simulink model "Test_Pattern_Generator"  (R2013b)
settings: Solver=ode45  StartTime=0.0  StopTime=1500  RelTol=1e-3
InitFcn:
  | %% DSPBuilder Start
  | alt_dspbuilder_update_model(bdroot)
  | %% DSPBuilder End
libraries: allblocks_alteradspbuilder2 x106, simulink x4
(part 1 of 2)
settings Model: Creator=Given_Jiang  LastModifiedBy=Given_Jiang

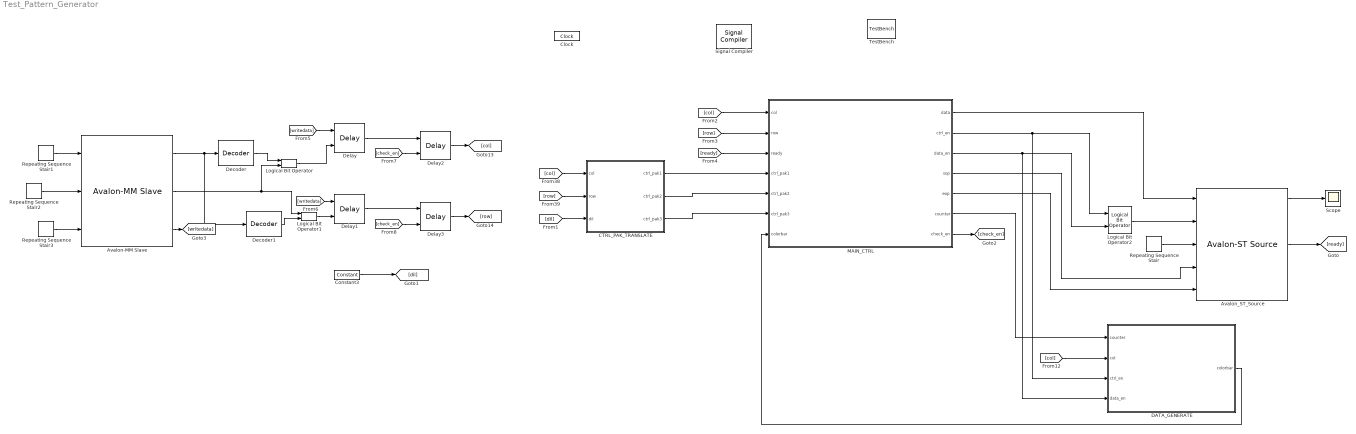
== system Test_Pattern_Generator ==
  Avalon-MM Slave : allblocks_alteradspbuilder2/Avalon-MM Slave  iofile=E:\FPGA\SOC\Quartus\quartus\dsp_builder\design\VIP_LIB\Test_Pattern_Generator\tb_Test_Pattern_Generator\Test%5FPattern%5FGenerator_Avalon-MM+Slave_address.salt,E:\FPGA\SOC\Quartus\quartus\dsp_builder\design\VIP_LIB\Test_Pattern_Generator\tb_Test_Pattern_Generator\Test%5FPattern%5FGenerator_Avalon-MM+Slave_write.salt,E:\FPGA\SOC\Quartus\quartus\dsp_builder\design\VIP_LIB\Test_Pattern_Generator\tb_Test_Pattern_Generator\Test%5FPattern%5FGenerator_Avalon-MM+Slave_writedata.salt,  SpecifyClock=off  addrWidth=2  addrAlignment=Dynamic  addrType=Write  BusType=Unsigned Integer  bwl=32  bwr=0  byteEnable=off  flowCtrl=off  pipeline=off  waitStateFormat=Fixed  readWaitStateCycles=0  writeWaitStateCycles=1  readLatencyFormat=Fixed  readLatencyCycles=0  burst=off  maxBurst=4  irq=off  receiveBeginTransfer=off  useChipSelect=off  externalType=Inferred  PORTTYPE=Output
  Avalon_ST_Source : allblocks_alteradspbuilder2/Avalon-ST Source  iofile=E:\FPGA\SOC\Quartus\quartus\dsp_builder\design\VIP_LIB\Test_Pattern_Generator\tb_Test_Pattern_Generator\Test%5FPattern%5FGenerator_Avalon%5FST%5FSource_data.capture,E:\FPGA\SOC\Quartus\quartus\dsp_builder\design\VIP_LIB\Test_Pattern_Generator\tb_Test_Pattern_Generator\Test%5FPattern%5FGenerator_Avalon%5FST%5FSource_valid.capture,E:\FPGA\SOC\Quartus\quartus\dsp_builder\design\VIP_LIB\Test_Pattern_Generator\tb_Test_Pattern_Generator\Test%5FPattern%5FGenerator_Avalon%5FST%5FSource_ready.salt,E:\FPGA\SOC\Quartus\quartus\dsp_builder\design\VIP_LIB\Test_Pattern_Generator\tb_Test_Pattern_Generator\Test%5FPattern%5FGenerator_Avalon%5FST%5FSource_startofpacket.capture,E:\FPGA\SOC\Quartus\quartus\dsp_builder\design\VIP_LIB\Test_Pattern_Generator\tb_Test_Pattern_Generator\Test%5FPattern%5FGenerator_Avalon%5FST%5FSource_endofpacket.capture,  SpecifyClock=off  BusType=Unsigned Integer  bwl=24  bwr=0  symbolWidth=8  symbolsPerBeat=3  numOfChannels=0  numOfErrorDescriptors=0  endOfPacket=on  startOfPacket=on  empty=off  readyLatency=1  externalType=Inferred  PORTTYPE=Input
  CTRL_PAK_TRANSLATE : Subsystem
  Clock : allblocks_alteradspbuilder2/Clock  ClockPeriod=7.5  ClockPeriodUnit=ns  SampleTime=1  ResetLatency=0  ResetRegisterCascadeDepth=0  SimulationStartCycle=5  PhaseOffset=0  Reset=aclr  ResetType=Active Low  Export=off
  Constant3 : allblocks_alteradspbuilder2/Constant  mask_cst=0  BusType=Signed Integer  bwl=4  bwr=0  roundMode=Truncate  satMode=Wrap  SpecifyClock=off  allowFloatingPointOverride=on  logOutputs=off  logFile=E:\FPGA\SOC\Quartus\quartus\dsp_builder\design\VIP_LIB\Test_Pattern_Generator\tb_Test_Pattern_Generator\Test%5FPattern%5FGenerator_Constant3.fixedpointlog
  DATA_GENERATE : Subsystem
  Decoder : allblocks_alteradspbuilder2/Decoder  BusType=Unsigned Integer  bwl=2  bwr=2  registered=on  pipeline_display=1  value=1
  Decoder1 : allblocks_alteradspbuilder2/Decoder  BusType=Unsigned Integer  bwl=2  bwr=2  registered=on  pipeline_display=1  value=2
  Delay : allblocks_alteradspbuilder2/Delay  pipeline=1  pipeline_display=1  ClockPhase=1  use_ena=on  use_sclr=off  allowFloatingPointOverride=on  logOutputs=off  logFile=E:\FPGA\SOC\Quartus\quartus\dsp_builder\design\VIP_LIB\Test_Pattern_Generator\tb_Test_Pattern_Generator\Test%5FPattern%5FGenerator_Delay.fixedpointlog  use_init=on  reset_value=32
  Delay1 : allblocks_alteradspbuilder2/Delay  pipeline=1  pipeline_display=1  ClockPhase=1  use_ena=on  use_sclr=off  allowFloatingPointOverride=on  logOutputs=off  logFile=E:\FPGA\SOC\Quartus\quartus\dsp_builder\design\VIP_LIB\Test_Pattern_Generator\tb_Test_Pattern_Generator\Test%5FPattern%5FGenerator_Delay1.fixedpointlog  use_init=on  reset_value=32
  Delay2 : allblocks_alteradspbuilder2/Delay  pipeline=1  pipeline_display=1  ClockPhase=1  use_ena=on  use_sclr=off  allowFloatingPointOverride=on  logOutputs=off  logFile=E:\FPGA\SOC\Quartus\quartus\dsp_builder\design\VIP_LIB\Test_Pattern_Generator\tb_Test_Pattern_Generator\Test%5FPattern%5FGenerator_Delay2.fixedpointlog  use_init=on  reset_value=32
  Delay3 : allblocks_alteradspbuilder2/Delay  pipeline=1  pipeline_display=1  ClockPhase=1  use_ena=on  use_sclr=off  allowFloatingPointOverride=on  logOutputs=off  logFile=E:\FPGA\SOC\Quartus\quartus\dsp_builder\design\VIP_LIB\Test_Pattern_Generator\tb_Test_Pattern_Generator\Test%5FPattern%5FGenerator_Delay3.fixedpointlog  use_init=on  reset_value=32
  Logical Bit Operator : allblocks_alteradspbuilder2/Logical Bit Operator  LogicalOperator=AND  user_inputs=2  pipeline_display=0
  Logical Bit Operator1 : allblocks_alteradspbuilder2/Logical Bit Operator  LogicalOperator=AND  user_inputs=2  pipeline_display=0
  Logical Bit Operator2 : allblocks_alteradspbuilder2/Logical Bit Operator  LogicalOperator=OR  user_inputs=2  pipeline_display=0
  MAIN_CTRL : Subsystem
  Repeating Sequence Stair : simulink/Sources/Repeating Sequence Stair  OutValues=[0 1 1 1 1 1 1].'  tsamp=-1  OutMin=[]  OutMax=[]  OutDataTypeStr=double  OutputDataTypeScalingMode=double  OutDataType=fixdt(0,8)  ConRadixGroup=Best Precision: Vector-wise  OutScaling=2^-12
  Repeating Sequence Stair1 : simulink/Sources/Repeating Sequence Stair  OutValues=[1].'  tsamp=-1  OutMin=[]  OutMax=[]  OutDataTypeStr=double  OutputDataTypeScalingMode=double  OutDataType=fixdt(0,8)  ConRadixGroup=Best Precision: Vector-wise  OutScaling=2^-12
  Repeating Sequence Stair2 : simulink/Sources/Repeating Sequence Stair  OutValues=[1].'  tsamp=-1  OutMin=[]  OutMax=[]  OutDataTypeStr=double  OutputDataTypeScalingMode=double  OutDataType=fixdt(0,8)  ConRadixGroup=Best Precision: Vector-wise  OutScaling=2^-12
  Repeating Sequence Stair3 : simulink/Sources/Repeating Sequence Stair  OutValues=[255].'  tsamp=-1  OutMin=[]  OutMax=[]  OutDataTypeStr=double  OutputDataTypeScalingMode=double  OutDataType=fixdt(0,8)  ConRadixGroup=Best Precision: Vector-wise  OutScaling=2^-12
  Scope : Scope
  Signal Compiler : allblocks_alteradspbuilder2/Signal Compiler  DeviceFamily=Cyclone V  DeviceName=AUTO  DisableEarlyHDLGeneration=off  EnableSignalTap=off  SignalTapDepth=128  UseBoardBlock=off  StpUseDefaultClock=on  StpClock=Clock  ExportDir=E:\FPGA\SOC\Quartus\quartus\dsp_builder
  TestBench : allblocks_alteradspbuilder2/TestBench  enable=on  advancedMode=on  modelSimGui=off  maxDisplayErrors=10  mismatchErrorLevel=Error  simdatafile=E:\FPGA\SOC\Quartus\quartus\dsp_builder\design\VIP_LIB\Test_Pattern_Generator\tb_Test_Pattern_Generator\Test_Pattern_Generator.simdata.tcl
  wires:
  Avalon_ST_Source/3 -> [ready]
  Logical Bit Operator2/1 -> Avalon_ST_Source/2
  MAIN_CTRL/4(sop) -> Avalon_ST_Source/4
  MAIN_CTRL/5(eop) -> Avalon_ST_Source/5
  [row] -> CTRL_PAK_TRANSLATE/2(row)
  [col] -> CTRL_PAK_TRANSLATE/1(col)
  [dil] -> CTRL_PAK_TRANSLATE/3(dil)
  Constant3/1 -> [dil]
  [col] -> MAIN_CTRL/1(col)
  [row] -> MAIN_CTRL/2(row)
  [ready] -> MAIN_CTRL/3(ready)
  CTRL_PAK_TRANSLATE/1(ctrl_pak1) -> MAIN_CTRL/4(ctrl_pak1)
  CTRL_PAK_TRANSLATE/2(ctrl_pak2) -> MAIN_CTRL/5(ctrl_pak2)
  CTRL_PAK_TRANSLATE/3(ctrl_pak3) -> MAIN_CTRL/6(ctrl_pak3)
  [col] -> DATA_GENERATE/2(col)
  DATA_GENERATE/1(colorbar) -> MAIN_CTRL/7(colorbar)
  MAIN_CTRL/6(counter) -> DATA_GENERATE/1(counter)
  MAIN_CTRL/3(data_en) -> DATA_GENERATE/4(data_en), Logical Bit Operator2/2
  MAIN_CTRL/2(ctrl_en) -> DATA_GENERATE/3(ctrl_en), Logical Bit Operator2/1
  MAIN_CTRL/1(data) -> Avalon_ST_Source/1
  Repeating Sequence Stair/1 -> Avalon_ST_Source/3
  MAIN_CTRL/7(check_en) -> [check_en]
  Logical Bit Operator/1 -> Delay/2
  Delay/1 -> Delay2/1
  [check_en] -> Delay2/2
  [check_en] -> Delay3/2
  Delay1/1 -> Delay3/1
  Delay2/1 -> [col]
  Delay3/1 -> [row]
  Avalon_ST_Source/1 -> Scope/1
  Repeating Sequence Stair1/1 -> Avalon-MM Slave/1
  Repeating Sequence Stair3/1 -> Avalon-MM Slave/3
  Avalon-MM Slave/1 -> Decoder1/1, Decoder/1
  Decoder/1 -> Logical Bit Operator/1
  Avalon-MM Slave/2 -> Logical Bit Operator1/1, Logical Bit Operator/2
  Decoder1/1 -> Logical Bit Operator1/2
  Logical Bit Operator1/1 -> Delay1/2
  Avalon-MM Slave/3 -> [writedata]
  [writedata] -> Delay/1
  [writedata] -> Delay1/1
  Repeating Sequence Stair2/1 -> Avalon-MM Slave/2

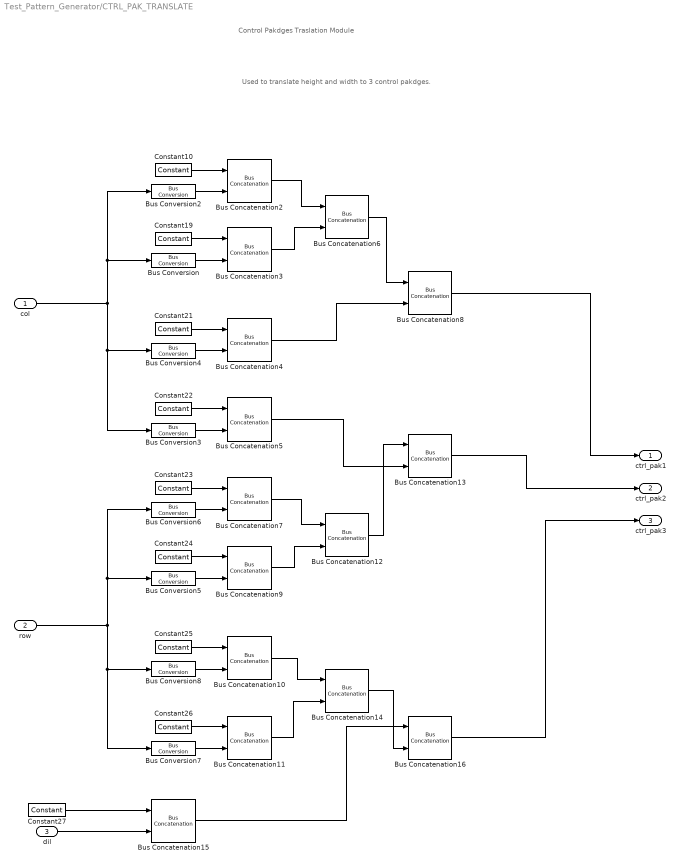
== system Test_Pattern_Generator/CTRL_PAK_TRANSLATE ==
  note: Used to translate height and width to 3 control pakdges.
  note: Control Pakdges Traslation Module
  col : Inport
  row : Inport  Port=2
  dil : Inport  Port=3
  Bus Concatenation{2..5,7,9..11,15} (9 alike) : allblocks_alteradspbuilder2/Bus Concatenation  isSigned=off  awidth=4  bwidth=4  pipeline_display=0
  Bus Concatenation12 : allblocks_alteradspbuilder2/Bus Concatenation  isSigned=off  awidth=8  bwidth=8  pipeline_display=0
  Bus Concatenation13 : allblocks_alteradspbuilder2/Bus Concatenation  isSigned=off  awidth=16  bwidth=8  pipeline_display=0
  Bus Concatenation14 : allblocks_alteradspbuilder2/Bus Concatenation  isSigned=off  awidth=8  bwidth=8  pipeline_display=0
  Bus Concatenation16 : allblocks_alteradspbuilder2/Bus Concatenation  isSigned=off  awidth=8  bwidth=16  pipeline_display=0
  Bus Concatenation6 : allblocks_alteradspbuilder2/Bus Concatenation  isSigned=off  awidth=8  bwidth=8  pipeline_display=0
  Bus Concatenation8 : allblocks_alteradspbuilder2/Bus Concatenation  isSigned=off  awidth=16  bwidth=8  pipeline_display=0
  Bus Conversion : allblocks_alteradspbuilder2/Bus Conversion  BusType=Unsigned Integer  ibwl=16  ibwr=1  bwl=4  bwr=1  bitToConnectToOutputLSB=8  round=off  saturate=off  pipeline_display=0
  Bus Conversion2 : allblocks_alteradspbuilder2/Bus Conversion  BusType=Unsigned Integer  ibwl=16  ibwr=1  bwl=4  bwr=1  bitToConnectToOutputLSB=4  round=off  saturate=off  pipeline_display=0
  Bus Conversion3 : allblocks_alteradspbuilder2/Bus Conversion  BusType=Unsigned Integer  ibwl=16  ibwr=1  bwl=4  bwr=1  bitToConnectToOutputLSB=0  round=off  saturate=off  pipeline_display=0
  Bus Conversion4 : allblocks_alteradspbuilder2/Bus Conversion  BusType=Unsigned Integer  ibwl=16  ibwr=1  bwl=4  bwr=1  bitToConnectToOutputLSB=12  round=off  saturate=off  pipeline_display=0
  Bus Conversion5 : allblocks_alteradspbuilder2/Bus Conversion  BusType=Unsigned Integer  ibwl=16  ibwr=1  bwl=4  bwr=1  bitToConnectToOutputLSB=12  round=off  saturate=off  pipeline_display=0
  Bus Conversion6 : allblocks_alteradspbuilder2/Bus Conversion  BusType=Unsigned Integer  ibwl=16  ibwr=1  bwl=4  bwr=1  bitToConnectToOutputLSB=8  round=off  saturate=off  pipeline_display=0
  Bus Conversion7 : allblocks_alteradspbuilder2/Bus Conversion  BusType=Unsigned Integer  ibwl=16  ibwr=1  bwl=4  bwr=1  bitToConnectToOutputLSB=4  round=off  saturate=off  pipeline_display=0
  Bus Conversion8 : allblocks_alteradspbuilder2/Bus Conversion  BusType=Unsigned Integer  ibwl=16  ibwr=1  bwl=4  bwr=1  bitToConnectToOutputLSB=0  round=off  saturate=off  pipeline_display=0
  Constant10 : allblocks_alteradspbuilder2/Constant  mask_cst=0  BusType=Signed Integer  bwl=4  bwr=0  roundMode=Truncate  satMode=Wrap  SpecifyClock=off  allowFloatingPointOverride=on  logOutputs=off  logFile=E:\FPGA\SOC\Quartus\quartus\dsp_builder\design\VIP_LIB\Test_Pattern_Generator\tb_Test_Pattern_Generator\Test%5FPattern%5FGenerator_CTRL%5FPAK%5FTRANSLATE_Constant10.fixedpointlog
  Constant19 : allblocks_alteradspbuilder2/Constant  mask_cst=0  BusType=Signed Integer  bwl=4  bwr=0  roundMode=Truncate  satMode=Wrap  SpecifyClock=off  allowFloatingPointOverride=on  logOutputs=off  logFile=E:\FPGA\SOC\Quartus\quartus\dsp_builder\design\VIP_LIB\Test_Pattern_Generator\tb_Test_Pattern_Generator\Test%5FPattern%5FGenerator_CTRL%5FPAK%5FTRANSLATE_Constant19.fixedpointlog
  Constant21 : allblocks_alteradspbuilder2/Constant  mask_cst=0  BusType=Signed Integer  bwl=4  bwr=0  roundMode=Truncate  satMode=Wrap  SpecifyClock=off  allowFloatingPointOverride=on  logOutputs=off  logFile=E:\FPGA\SOC\Quartus\quartus\dsp_builder\design\VIP_LIB\Test_Pattern_Generator\tb_Test_Pattern_Generator\Test%5FPattern%5FGenerator_CTRL%5FPAK%5FTRANSLATE_Constant21.fixedpointlog
  Constant22 : allblocks_alteradspbuilder2/Constant  mask_cst=0  BusType=Signed Integer  bwl=4  bwr=0  roundMode=Truncate  satMode=Wrap  SpecifyClock=off  allowFloatingPointOverride=on  logOutputs=off  logFile=E:\FPGA\SOC\Quartus\quartus\dsp_builder\design\VIP_LIB\Test_Pattern_Generator\tb_Test_Pattern_Generator\Test%5FPattern%5FGenerator_CTRL%5FPAK%5FTRANSLATE_Constant22.fixedpointlog
  Constant23 : allblocks_alteradspbuilder2/Constant  mask_cst=0  BusType=Signed Integer  bwl=4  bwr=0  roundMode=Truncate  satMode=Wrap  SpecifyClock=off  allowFloatingPointOverride=on  logOutputs=off  logFile=E:\FPGA\SOC\Quartus\quartus\dsp_builder\design\VIP_LIB\Test_Pattern_Generator\tb_Test_Pattern_Generator\Test%5FPattern%5FGenerator_CTRL%5FPAK%5FTRANSLATE_Constant23.fixedpointlog
  Constant24 : allblocks_alteradspbuilder2/Constant  mask_cst=0  BusType=Signed Integer  bwl=4  bwr=0  roundMode=Truncate  satMode=Wrap  SpecifyClock=off  allowFloatingPointOverride=on  logOutputs=off  logFile=E:\FPGA\SOC\Quartus\quartus\dsp_builder\design\VIP_LIB\Test_Pattern_Generator\tb_Test_Pattern_Generator\Test%5FPattern%5FGenerator_CTRL%5FPAK%5FTRANSLATE_Constant24.fixedpointlog
  Constant25 : allblocks_alteradspbuilder2/Constant  mask_cst=0  BusType=Signed Integer  bwl=4  bwr=0  roundMode=Truncate  satMode=Wrap  SpecifyClock=off  allowFloatingPointOverride=on  logOutputs=off  logFile=E:\FPGA\SOC\Quartus\quartus\dsp_builder\design\VIP_LIB\Test_Pattern_Generator\tb_Test_Pattern_Generator\Test%5FPattern%5FGenerator_CTRL%5FPAK%5FTRANSLATE_Constant25.fixedpointlog
  Constant26 : allblocks_alteradspbuilder2/Constant  mask_cst=0  BusType=Signed Integer  bwl=4  bwr=0  roundMode=Truncate  satMode=Wrap  SpecifyClock=off  allowFloatingPointOverride=on  logOutputs=off  logFile=E:\FPGA\SOC\Quartus\quartus\dsp_builder\design\VIP_LIB\Test_Pattern_Generator\tb_Test_Pattern_Generator\Test%5FPattern%5FGenerator_CTRL%5FPAK%5FTRANSLATE_Constant26.fixedpointlog
  Constant27 : allblocks_alteradspbuilder2/Constant  mask_cst=0  BusType=Signed Integer  bwl=4  bwr=0  roundMode=Truncate  satMode=Wrap  SpecifyClock=off  allowFloatingPointOverride=on  logOutputs=off  logFile=E:\FPGA\SOC\Quartus\quartus\dsp_builder\design\VIP_LIB\Test_Pattern_Generator\tb_Test_Pattern_Generator\Test%5FPattern%5FGenerator_CTRL%5FPAK%5FTRANSLATE_Constant27.fixedpointlog
  ctrl_pak1 : Outport
  ctrl_pak2 : Outport  Port=2
  ctrl_pak3 : Outport  Port=3
  wires:
  col/1 -> Bus Conversion3/1, Bus Conversion4/1, Bus Conversion2/1, Bus Conversion/1
  Bus Conversion2/1 -> Bus Concatenation2/2
  Constant10/1 -> Bus Concatenation2/1
  Constant19/1 -> Bus Concatenation3/1
  Bus Conversion/1 -> Bus Concatenation3/2
  Constant21/1 -> Bus Concatenation4/1
  Bus Conversion4/1 -> Bus Concatenation4/2
  Constant22/1 -> Bus Concatenation5/1
  Bus Conversion3/1 -> Bus Concatenation5/2
  Bus Concatenation3/1 -> Bus Concatenation6/2
  Bus Concatenation4/1 -> Bus Concatenation8/2
  Bus Concatenation6/1 -> Bus Concatenation8/1
  row/1 -> Bus Conversion7/1, Bus Conversion8/1, Bus Conversion6/1, Bus Conversion5/1
  Bus Conversion6/1 -> Bus Concatenation7/2
  Constant23/1 -> Bus Concatenation7/1
  Constant24/1 -> Bus Concatenation9/1
  Bus Conversion5/1 -> Bus Concatenation9/2
  Constant25/1 -> Bus Concatenation10/1
  Bus Conversion8/1 -> Bus Concatenation10/2
  Constant26/1 -> Bus Concatenation11/1
  Bus Conversion7/1 -> Bus Concatenation11/2
  Bus Concatenation7/1 -> Bus Concatenation12/1
  Bus Concatenation9/1 -> Bus Concatenation12/2
  Bus Concatenation10/1 -> Bus Concatenation14/1
  Bus Concatenation11/1 -> Bus Concatenation14/2
  dil/1 -> Bus Concatenation15/2
  Constant27/1 -> Bus Concatenation15/1
  Bus Concatenation8/1 -> ctrl_pak1/1
  Bus Concatenation13/1 -> ctrl_pak2/1
  Bus Concatenation16/1 -> ctrl_pak3/1
  Bus Concatenation2/1 -> Bus Concatenation6/1
  Bus Concatenation5/1 -> Bus Concatenation13/2
  Bus Concatenation12/1 -> Bus Concatenation13/1
  Bus Concatenation15/1 -> Bus Concatenation16/1
  Bus Concatenation14/1 -> Bus Concatenation16/2

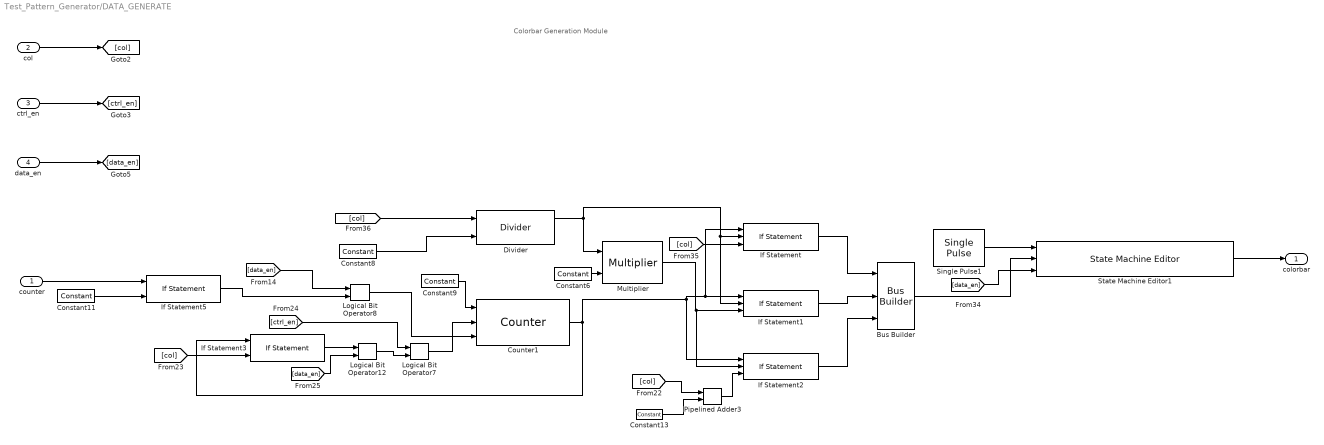
== system Test_Pattern_Generator/DATA_GENERATE ==
  note: Colorbar Generation Module
  counter : Inport
  col : Inport  Port=2
  ctrl_en : Inport  Port=3
  data_en : Inport  Port=4
  Bus Builder : allblocks_alteradspbuilder2/Bus Builder  BusType=Unsigned Integer  bwl=3  bwr=1  pipeline_display=0
  Constant11 : allblocks_alteradspbuilder2/Constant  mask_cst=4  BusType=Unsigned Integer  bwl=16  bwr=0  roundMode=Truncate  satMode=Wrap  SpecifyClock=off  allowFloatingPointOverride=on  logOutputs=off  logFile=E:\FPGA\SOC\Quartus\quartus\dsp_builder\design\VIP_LIB\Test_Pattern_Generator\tb_Test_Pattern_Generator\Test%5FPattern%5FGenerator_DATA%5FGENERATE_Constant11.fixedpointlog
  Constant13 : allblocks_alteradspbuilder2/Constant  mask_cst=1  BusType=Unsigned Integer  bwl=24  bwr=0  roundMode=Truncate  satMode=Wrap  SpecifyClock=off  allowFloatingPointOverride=on  logOutputs=off  logFile=E:\FPGA\SOC\Quartus\quartus\dsp_builder\design\VIP_LIB\Test_Pattern_Generator\tb_Test_Pattern_Generator\Test%5FPattern%5FGenerator_DATA%5FGENERATE_Constant13.fixedpointlog
  Constant6 : allblocks_alteradspbuilder2/Constant  mask_cst=2  BusType=Unsigned Integer  bwl=24  bwr=0  roundMode=Truncate  satMode=Wrap  SpecifyClock=off  allowFloatingPointOverride=on  logOutputs=off  logFile=E:\FPGA\SOC\Quartus\quartus\dsp_builder\design\VIP_LIB\Test_Pattern_Generator\tb_Test_Pattern_Generator\Test%5FPattern%5FGenerator_DATA%5FGENERATE_Constant6.fixedpointlog
  Constant8 : allblocks_alteradspbuilder2/Constant  mask_cst=3  BusType=Unsigned Integer  bwl=24  bwr=0  roundMode=Truncate  satMode=Wrap  SpecifyClock=off  allowFloatingPointOverride=on  logOutputs=off  logFile=E:\FPGA\SOC\Quartus\quartus\dsp_builder\design\VIP_LIB\Test_Pattern_Generator\tb_Test_Pattern_Generator\Test%5FPattern%5FGenerator_DATA%5FGENERATE_Constant8.fixedpointlog
  Constant9 : allblocks_alteradspbuilder2/Constant  mask_cst=1  BusType=Unsigned Integer  bwl=24  bwr=0  roundMode=Truncate  satMode=Wrap  SpecifyClock=off  allowFloatingPointOverride=on  logOutputs=off  logFile=E:\FPGA\SOC\Quartus\quartus\dsp_builder\design\VIP_LIB\Test_Pattern_Generator\tb_Test_Pattern_Generator\Test%5FPattern%5FGenerator_DATA%5FGENERATE_Constant9.fixedpointlog
  Counter1 : allblocks_alteradspbuilder2/Counter  BusType=Unsigned Integer  bwl=24  bwr=0  use_modulo=on  modulo=2^16  SpecifyClock=off  direction=Increment  use_sload=on  use_sset=off  svalue=1  use_clk_ena=off  use_ena=on  use_sclr=off  pipeline_display=1
  Divider : allblocks_alteradspbuilder2/Divider  BusType=Unsigned Integer  bwl=24  bwr=0  pipeline=0  pipeline_display=0  use_ena=off  use_aclr=off
  If Statement : allblocks_alteradspbuilder2/If Statement  user_inputs=3  if_expression=((a>0)&(a<b))|(a=c)  BusType=Unsigned Integer  bwl=24  bwr=0  pipeline_display=1  use_else_output=off  use_elseif_input=off
  If Statement1 : allblocks_alteradspbuilder2/If Statement  user_inputs=3  if_expression=((a>b)|(a=b))&(a<c)  BusType=Unsigned Integer  bwl=24  bwr=0  pipeline_display=1  use_else_output=off  use_elseif_input=off
  If Statement2 : allblocks_alteradspbuilder2/If Statement  user_inputs=3  if_expression=((a>b)|(a=b))&((a<c)|(a=c))  BusType=Unsigned Integer  bwl=24  bwr=0  pipeline_display=1  use_else_output=off  use_elseif_input=off
  If Statement3 : allblocks_alteradspbuilder2/If Statement  user_inputs=2  if_expression=a=b  BusType=Unsigned Integer  bwl=24  bwr=0  pipeline_display=1  use_else_output=off  use_elseif_input=off
  If Statement5 : allblocks_alteradspbuilder2/If Statement  user_inputs=2  if_expression=a>b  BusType=Unsigned Integer  bwl=24  bwr=0  pipeline_display=1  use_else_output=off  use_elseif_input=off
  Logical Bit Operator12 : allblocks_alteradspbuilder2/Logical Bit Operator  LogicalOperator=AND  user_inputs=2  pipeline_display=0
  Logical Bit Operator7 : allblocks_alteradspbuilder2/Logical Bit Operator  LogicalOperator=OR  user_inputs=2  pipeline_display=0
  Logical Bit Operator8 : allblocks_alteradspbuilder2/Logical Bit Operator  LogicalOperator=AND  user_inputs=2  pipeline_display=0
  Multiplier : allblocks_alteradspbuilder2/Multiplier  BusType=Unsigned Integer  bwl=24  bwr=0  pipeline=0  pipeline_display=0  allowFloatingPointOverride=on  logOutputs=off  logFile=E:\FPGA\SOC\Quartus\quartus\dsp_builder\design\VIP_LIB\Test_Pattern_Generator\tb_Test_Pattern_Generator\Test%5FPattern%5FGenerator_DATA%5FGENERATE_Multiplier.fixedpointlog  UseEqualInputWidth=on  bbwl=8  bbwr=0  FullResolution=on  OutputMsb=8  OutputLsb=0  OutputBwl=16  OutputBwr=16  UseDedicatedCircuitry=YES  use_ena=off  use_aclr=off
  Pipelined Adder3 : allblocks_alteradspbuilder2/Pipelined Adder  BusType=Unsigned Integer  bwl=24  bwr=0  pipeline=2  pipeline_display=2  AddSubDirection=SUB  use_cin=off  use_ovl=off  use_addsub=off  use_ena=off  use_aclr=off  or_aclr_inputs=on
  Single Pulse1 : allblocks_alteradspbuilder2/Single Pulse  signal_type=Step Down  impulse_width=1  delay=1  SpecifyClock=off  use_ena=off  use_sclr=off
  State Machine Editor1 : allblocks_alteradspbuilder2/State Machine Editor  entityName=StateMachineEditor1_import  use_dynamic_feedthrough_data=on  inNames=reset col_select data_en  inBwls=1 3 1  inBwrs="0  0  0"  inTypes=b s b  inDelayed="0  1  1"  outNames=data  outBwls=24  outBwrs=0  outTypes=s  n_input_port=3  n_output_port=1  array_clocks=clock  xmlmapfile=E:\FPGA\SOC\Quartus\quartus\dsp_builder\lib\SimgenCMap.xml  vofile=DSPBuilder_Test_Pattern_Generator_import\StateMachineEditor1.vo  use_systemC_model=off  is_megacore=off  smf_variation=|
      | /*                                                                         
      | WARNING: Do NOT edit the input and output ports in this file in a text     
      | editor if you plan to continue editing the block that represents it in     
      | the Block Editor! File corruption is VERY likely to occur.                 
      | Copyright (C) 1991-2013 Altera Corporation                                 
      | Your use of Altera Corporation's design tools, logic functions             
      | and other software and tools, and its AMPP partner logic                   
      | functions, and any output files from any of the foregoing                  
      | (including device programming or simulation files), and any                
      | associated documentation or information are expressly subject              
      | to the terms and conditions of the Altera Program License                  
      | Subscription Agreement, Altera MegaCore Function License                   
      | Agreement, or other applicable license agreement, including,               
      | without limitation, that your use is for the sole purpose of               
      | programming logic devices manufactured by Altera and sold by               
      | Altera or its authorized distributors.  Please refer to the                
      | applicable agreement for further details.                                  
      | Generated by Quartus II Version 13.1.0 Build 162 10/23/2013 SJ Full Version
      | Created on Sat Feb 07 15:51:54 2015                                        
      | */                                                                         
      | VERSION = "3.0";                                                           
      | HEADER                                                                     
      | (                                                                          
      | 	GENERAL{                                                                  
      | 		RMODE = "S";                                                             
      | 		RA_LEVEL = "H";                                                          
      | 		HOPT = "VHDL";                                                           
      | 	}                                                                         
      | 	SPORT{                                                                    
      | 		NAME = "clock";                                                          
      | 		PTYPE = "CI";                                                            
      | 		REG = "N";                                                               
      | 		OUTS = "N";                                                              
      | 	}                                                                         
      | 	SPORT{                                                                    
      | 		NAME = "reset";                                                          
      | 		PTYPE = "RI";                                                            
      | 		REG = "N";                                                               
      | 		OUTS = "N";                                                              
      | 	}                                                                         
      | 	SPORT{                                                                    
      | 		NAME = "col_select[2:0]";                                                
      | 		PTYPE = "OI";                                                            
      | 		REG = "N";                                                               
      | 		OUTS = "N";                                                              
      | 	}                                                                         
      | 	SPORT{                                                                    
      | 		NAME = "data_en";                                                        
      | 		PTYPE = "OI";                                                            
      | 		REG = "N";                                                               
      | 		OUTS = "N";                                                              
      | 	}                                                                         
      | 	SPORT{                                                                    
      | 		NAME = "data[23:0]";                                                     
      | 		PTYPE = "OU";                                                            
      | 		REG = "N";                                                               
      | 		OUTS = "C";                                                              
      | 	}                                                                         
      | 	STATE{                                                                    
      | 		NAME = "IDLE";                                                           
      | 		STYPE = "RE";                                                            
      | 		PT = (192,224);                                                          
      | 		OUTP = "data[23:0]";                                                     
      | 		OUT_VALUE = "0";                                                         
      | 		COND = "";                                                               
      | 	}                                                                         
      | 	STATE{                                                                    
      | 		NAME = "BLOCKA";                                                         
      | 		STYPE = "NR";                                                            
      | 		PT = (368,224);                                                          
      | 		OUTP = "data[23:0]";                                                     
      | 		OUT_VALUE = "255";                                                       
      | 		COND = "";                                                               
      | 	}                                                                         
      | 	STATE{                                                                    
      | 		NAME = "BLOCKB";                                                         
      | 		STYPE = "NR";                                                            
      | 		PT = (520,224);                                                          
      | 		OUTP = "data[23:0]";                                                     
      | 		OUT_VALUE = "65280";                                                     
      | 		COND = "";                                                               
      | 	}                                                                         
      | 	STATE{                                                                    
      | 		NAME = "BLOCKC";                                                         
      | 		STYPE = "NR";                                                            
      | 		PT = (680,224);                                                          
      | 		OUTP = "data[23:0]";                                                     
      | 		OUT_VALUE = "16711680";                                                  
      | 		COND = "";                                                               
      | 	}                                                                         
      | 	TRANS{                                                                    
      | 		SSTATE = "BLOCKC";                                                       
      | 		DSTATE = "IDLE";                                                         
      | 		EQ = "col_select==0";                                                    
      | 		PT = (689,268);                                                          
      | 		PT = (573,317);                                                          
      | 		PT = (364,317);                                                          
      | 		PT = (231,268);                                                          
      | 		PT = (468,327);                                                          
      | 	}                                                                         
      | 	TRANS{                                                                    
      | 		SSTATE = "IDLE";                                                         
      | 		DSTATE = "BLOCKA";                                                       
      | 		EQ = "(col_select==1)&(data_en==1)";                                     
      | 		PT = (241,248);                                                          
      | 		PT = (283,248);                                                          
      | 		PT = (325,248);                                                          
      | 		PT = (367,248);                                                          
      | 		PT = (304,258);                                                          
      | 	}                                                                         
      | 	TRANS{                                                                    
      | 		SSTATE = "BLOCKA";                                                       
      | 		DSTATE = "BLOCKB";                                                       
      | 		EQ = "(col_select==2)&(data_en==1)";                                     
      | 		PT = (417,248);                                                          
      | 		PT = (451,248);                                                          
      | 		PT = (485,248);                                                          
      | 		PT = (519,248);                                                          
      | 		PT = (468,258);                                                          
      | 	}                                                                         
      | 	TRANS{                                                                    
      | 		SSTATE = "BLOCKB";                                                       
      | 		DSTATE = "BLOCKC";                                                       
      | 		EQ = "(col_select==4)&(data_en==1)";                                     
      | 		PT = (569,248);                                                          
      | 		PT = (605,248);                                                          
      | 		PT = (642,248);                                                          
      | 		PT = (679,248);                                                          
      | 		PT = (601,249);                                                          
      | 	}                                                                         
      | 	TRANS{                                                                    
      | 		SSTATE = "IDLE";                                                         
      | 		DSTATE = "IDLE";                                                         
      | 		EQ = "col_select==0";                                                    
      | 		PT = (234,231);                                                          
      | 		PT = (270,231);                                                          
      | 		PT = (270,266);                                                          
      | 		PT = (234,266);                                                          
      | 		PT = (275,246);                                                          
      | 	}                                                                         
      | 	TRANS{                                                                    
      | 		SSTATE = "BLOCKC";                                                       
      | 		DSTATE = "BLOCKA";                                                       
      | 		EQ = "(col_select==1)&(data_en==1)";                                     
      | 		PT = (689,268);                                                          
      | 		PT = (587,321);                                                          
      | 		PT = (474,276);                                                          
      | 		PT = (407,268);                                                          
      | 		PT = (596,293);                                                          
      | 	}                                                                         
      | )                                                                          
      | END
  colorbar : Outport
  wires:
  Single Pulse1/1 -> State Machine Editor1/1
  Counter1/1 -> If Statement3/1, If Statement/1, If Statement1/1, If Statement2/1
  If Statement/1 -> Bus Builder/1
  If Statement1/1 -> Bus Builder/2
  If Statement2/1 -> Bus Builder/3
  Bus Builder/1 -> State Machine Editor1/2
  [col] -> Divider/1
  Constant8/1 -> Divider/2
  Constant6/1 -> Multiplier/2
  Constant9/1 -> Counter1/1
  Divider/1 -> Multiplier/1, If Statement/2, If Statement1/2
  Multiplier/1 -> If Statement2/2, If Statement1/3
  Logical Bit Operator7/1 -> Counter1/2
  counter/1 -> If Statement5/1
  Constant11/1 -> If Statement5/2
  [ctrl_en] -> Logical Bit Operator7/1
  [data_en] -> Logical Bit Operator8/1
  If Statement5/1 -> Logical Bit Operator8/2
  Logical Bit Operator8/1 -> Counter1/3
  [data_en] -> State Machine Editor1/3
  [col] -> If Statement3/2
  If Statement3/1 -> Logical Bit Operator12/1
  [data_en] -> Logical Bit Operator12/2
  Logical Bit Operator12/1 -> Logical Bit Operator7/2
  [col] -> Pipelined Adder3/1
  Constant13/1 -> Pipelined Adder3/2
  Pipelined Adder3/1 -> If Statement2/3
  [col] -> If Statement/3
  col/1 -> [col]
  ctrl_en/1 -> [ctrl_en]
  data_en/1 -> [data_en]
  State Machine Editor1/1 -> colorbar/1

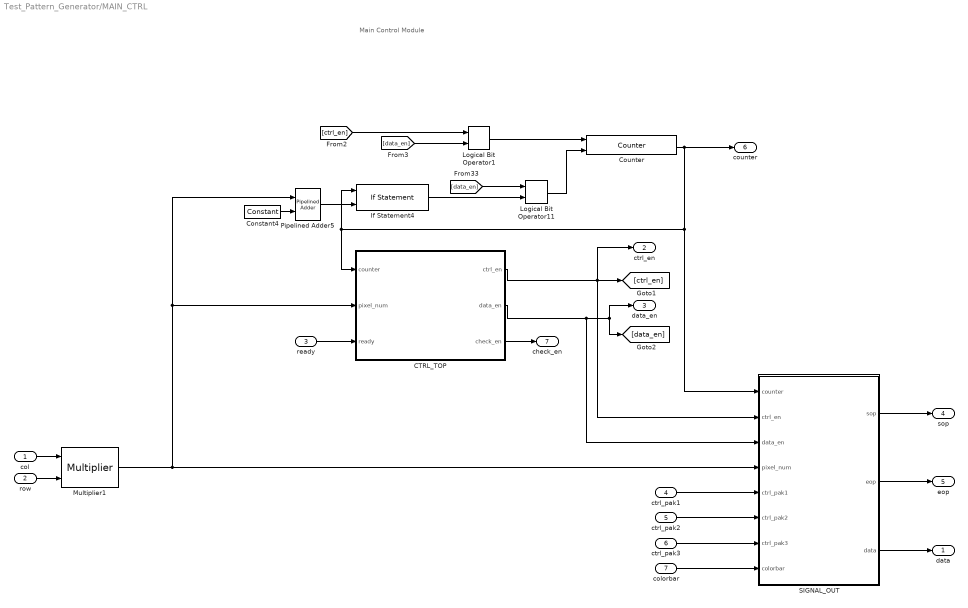
== system Test_Pattern_Generator/MAIN_CTRL ==
  note: Main Control Module
  col : Inport
  row : Inport  Port=2
  ready : Inport  Port=3
  ctrl_pak1 : Inport  Port=4
  ctrl_pak2 : Inport  Port=5
  ctrl_pak3 : Inport  Port=6
  colorbar : Inport  Port=7
  CTRL_TOP : Subsystem
  Constant4 : allblocks_alteradspbuilder2/Constant  mask_cst=4  BusType=Unsigned Integer  bwl=24  bwr=0  roundMode=Truncate  satMode=Wrap  SpecifyClock=off  allowFloatingPointOverride=on  logOutputs=off  logFile=E:\FPGA\SOC\Quartus\quartus\dsp_builder\design\VIP_LIB\Test_Pattern_Generator\tb_Test_Pattern_Generator\Test%5FPattern%5FGenerator_MAIN%5FCTRL_Constant4.fixedpointlog
  Counter : allblocks_alteradspbuilder2/Counter  BusType=Unsigned Integer  bwl=24  bwr=0  use_modulo=on  modulo=2^23  SpecifyClock=off  direction=Increment  use_sload=off  use_sset=off  svalue=1  use_clk_ena=off  use_ena=on  use_sclr=on  pipeline_display=1
  If Statement4 : allblocks_alteradspbuilder2/If Statement  user_inputs=2  if_expression=a=b  BusType=Unsigned Integer  bwl=24  bwr=0  pipeline_display=1  use_else_output=off  use_elseif_input=off
  Logical Bit Operator1 : allblocks_alteradspbuilder2/Logical Bit Operator  LogicalOperator=OR  user_inputs=2  pipeline_display=0
  Logical Bit Operator11 : allblocks_alteradspbuilder2/Logical Bit Operator  LogicalOperator=AND  user_inputs=2  pipeline_display=0
  Multiplier1 : allblocks_alteradspbuilder2/Multiplier  BusType=Unsigned Integer  bwl=24  bwr=0  pipeline=0  pipeline_display=0  allowFloatingPointOverride=on  logOutputs=off  logFile=E:\FPGA\SOC\Quartus\quartus\dsp_builder\design\VIP_LIB\Test_Pattern_Generator\tb_Test_Pattern_Generator\Test%5FPattern%5FGenerator_MAIN%5FCTRL_Multiplier1.fixedpointlog  UseEqualInputWidth=on  bbwl=8  bbwr=0  FullResolution=on  OutputMsb=8  OutputLsb=0  OutputBwl=16  OutputBwr=16  UseDedicatedCircuitry=YES  use_ena=off  use_aclr=off
  Pipelined Adder5 : allblocks_alteradspbuilder2/Pipelined Adder  BusType=Unsigned Integer  bwl=24  bwr=0  pipeline=0  pipeline_display=0  AddSubDirection=ADD  use_cin=off  use_ovl=off  use_addsub=off  use_ena=off  use_aclr=off  or_aclr_inputs=on
  SIGNAL_OUT : Subsystem
  data : Outport
  ctrl_en : Outport  Port=2
  data_en : Outport  Port=3
  sop : Outport  Port=4
  eop : Outport  Port=5
  counter : Outport  Port=6
  check_en : Outport  Port=7
  wires:
  col/1 -> Multiplier1/1
  row/1 -> Multiplier1/2
  Multiplier1/1 -> SIGNAL_OUT/4(pixel_num), CTRL_TOP/2(pixel_num), Pipelined Adder5/1
  ready/1 -> CTRL_TOP/3(ready)
  Counter/1 -> counter/1, SIGNAL_OUT/1(counter), CTRL_TOP/1(counter), If Statement4/1
  [ctrl_en] -> Logical Bit Operator1/1
  Logical Bit Operator1/1 -> Counter/1
  [data_en] -> Logical Bit Operator1/2
  Pipelined Adder5/1 -> If Statement4/2
  If Statement4/1 -> Logical Bit Operator11/2
  [data_en] -> Logical Bit Operator11/1
  Logical Bit Operator11/1 -> Counter/2
  Constant4/1 -> Pipelined Adder5/2
  SIGNAL_OUT/3(data) -> data/1
  colorbar/1 -> SIGNAL_OUT/8(colorbar)
  SIGNAL_OUT/1(sop) -> sop/1
  SIGNAL_OUT/2(eop) -> eop/1
  ctrl_pak1/1 -> SIGNAL_OUT/5(ctrl_pak1)
  ctrl_pak2/1 -> SIGNAL_OUT/6(ctrl_pak2)
  ctrl_pak3/1 -> SIGNAL_OUT/7(ctrl_pak3)
  CTRL_TOP/1(ctrl_en) -> ctrl_en/1, SIGNAL_OUT/2(ctrl_en), [ctrl_en]
  CTRL_TOP/2(data_en) -> SIGNAL_OUT/3(data_en), [data_en], data_en/1
  CTRL_TOP/3(check_en) -> check_en/1
